simulink model "sensorfusion"  (R2022b)
settings: Solver=VariableStepAuto  StartTime=0.0  StopTime=180  RelTol=1e-3
settings Model: Creator=soup1997  LastModifiedBy=soup1997

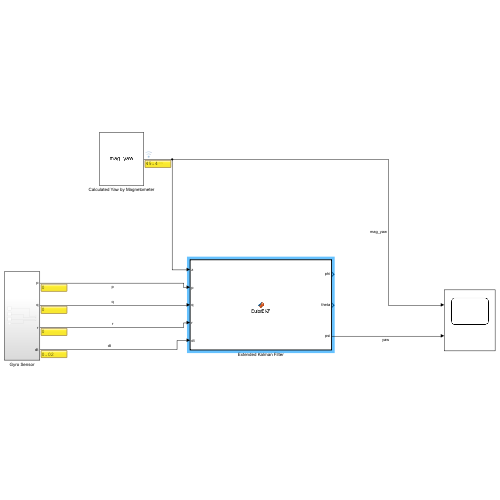
[thumbnail: Simulink's stored preview of the top-level diagram]
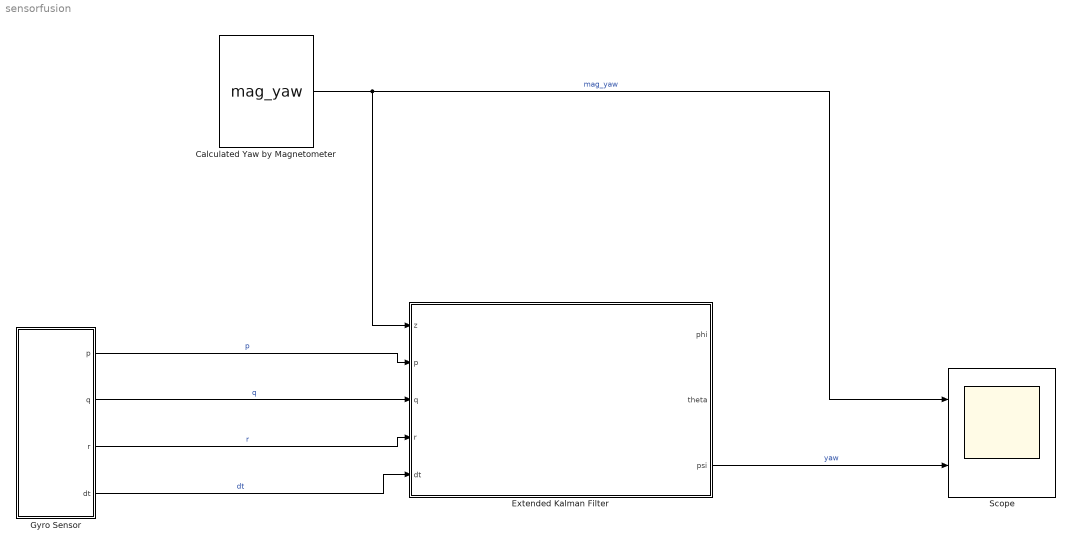
== system sensorfusion ==
  Calculated Yaw by Magnetometer : FromWorkspace  VariableName=mag_yaw  SampleTime=0.02
  Extended Kalman Filter : MATLAB Function  TreatAsAtomicUnit=on
  Gyro Sensor : Subsystem
  Scope : Scope  NumInputPorts=2
  wires:
  Gyro Sensor/1(p) -> Extended Kalman Filter/2(p)  "p"
  Gyro Sensor/2(q) -> Extended Kalman Filter/3(q)  "q"
  Gyro Sensor/3(r) -> Extended Kalman Filter/4(r)  "r"
  Gyro Sensor/4(dt) -> Extended Kalman Filter/5(dt)  "dt"
  Calculated Yaw by Magnetometer/1 -> Extended Kalman Filter/1(z), Scope/1  "mag_yaw"
  Extended Kalman Filter/3(psi) -> Scope/2  "yaw"

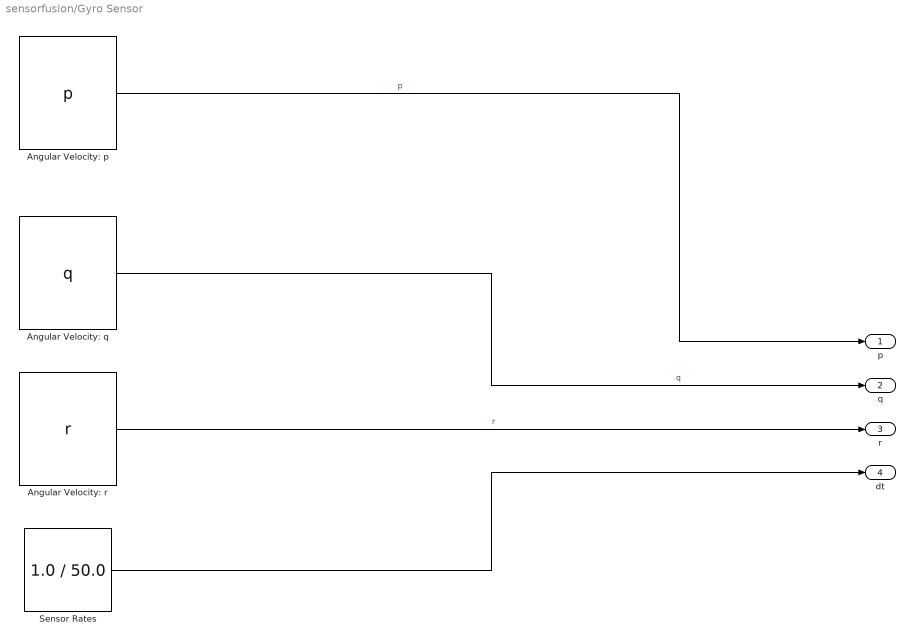
== system sensorfusion/Gyro Sensor ==
  Angular Velocity: p : FromWorkspace  VariableName=p  SampleTime=0.02
  Angular Velocity: q : FromWorkspace  VariableName=q  SampleTime=0.02
  Angular Velocity: r : FromWorkspace  VariableName=r  SampleTime=0.02
  Sensor Rates : Constant  Value=1.0 / 50.0
  p : Outport
  q : Outport  Port=2
  r : Outport  Port=3
  dt : Outport  Port=4
  wires:
  Angular Velocity: r/1 -> r/1  "r"
  Angular Velocity: p/1 -> p/1  "p"
  Angular Velocity: q/1 -> q/1  "q"
  Sensor Rates/1 -> dt/1

== matlab function sensorfusion/Extended Kalman Filter ==
  data: z input; phi output; p input; q input; r input; dt input; theta output; psi output
function [phi, theta, psi] = EulerEKF(z, p, q, r, dt)

persistent H Q R
persistent x_hat P
persistent firstRun


if isempty(firstRun)
    % accelerometer can't measure yaw rate
    H = diag([0, 0, 1]);
    
    % system noise
    Q = [0.0001, 0, 0;
         0, 0.0001, 0;
         0, 0, 0.1];
    
    % measurement noise
    R = diag([0, 0, 10]);

    x_hat = [0, 0, 0]'; % initial state variable(roll=0, pitch=0, yaw=0)

    P = 10.0 * eye(3); % initial covariance

    firstRun = 1;
end

A = Ajacob(x_hat, p, q, r, dt);

% step 1: Predict state & error covariance
xp = fx(x_hat, p, q, r, dt);
Pp = A*P*A' + Q;

% step 2: Compute Kalman gain
K = Pp*H' * pinv(H*Pp*H' + R);

% step 3: Compute the state estimate
x_hat = xp + K*(z - H*xp);

% step 4: Compute the error covariance
P = Pp - K*H*Pp;

phi = x_hat(1);
theta = x_hat(2);
psi = x_hat(3);

%------------------------
% function xp:
% Compute the angular velocity(p, q, r) to euler rate
% return predicted x
function xp = fx(xhat, p, q, r, dt)

phi = xhat(1);
theta = xhat(2);

xdot = zeros(3, 1);
xdot(1) = p + q*sin(phi)*tan(theta) + r*cos(phi)*tan(theta);
xdot(2) = q*cos(phi) - r*sin(phi);
xdot(3) = q*sin(phi)*sec(theta) + r*cos(phi)*sec(theta);

xp = xhat + xdot*dt; % cumulative sum

%------------------------
% function Ajacob:
% Compute the jacobian matrix of f(x)
% return A
function A = Ajacob(xhat, p, q, r, dt)

A = zeros(3, 3);
phi = xhat(1);
theta = xhat(2);

A(1, 1) = q*cos(phi)*tan(theta) - r*sin(phi)*tan(theta);
A(1, 2) = q*sin(phi)*sec(theta)^2 + r*cos(phi)*sec(theta)^2;
A(1, 3) = 0;

A(2, 1) = -q*sin(phi) - r*cos(phi);
A(2, 2) = 0;
A(2, 3) = 0;

A(3, 1) = q*cos(phi)*sec(theta) - r*sin(phi)*sec(theta);
A(3, 2) = q*sin(phi)*sec(theta)*tan(theta) + r*cos(phi)*sec(theta)*tan(theta);
A(3, 3) = 0;

A = eye(3) + A*dt;
